simulink model "my_simulink_demo"  (Simulink 7.9)
settings: Solver=FixedStepDiscrete  StartTime=0.0  StopTime=0.0  RelTol=1e-3
undefined symbols (not defined in the file or in its folder): jet
libraries: visionsinks x3, visionanalysis x1, visionsources x1, visiongeotforms x1
settings Model: Creator=lenovo  LastModifiedBy=lenovo

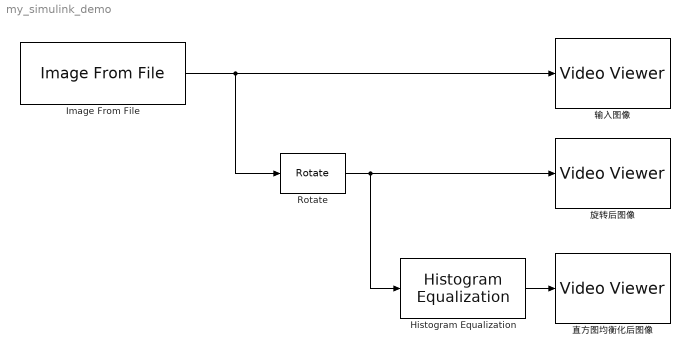
== system my_simulink_demo ==
  Histogram Equalization : visionanalysis/Histogram Equalization  specify=Uniform  numbins=64  src=Specify via dialog  hist=ones(1,64)
  Image From File : visionsources/Image From File  Tag=vipblks_nd  FileName=pout.tif  imagePorts=One multidimensional signal  Ts=inf  ImageDataType=Inherit from input image  Signed=on  WordLength=16  sdImageDataType=uint(8)  FractionLengthMode=User-defined  FractionLength=15  OutPortLabels=R|G|B
  Rotate : visiongeotforms/Rotate  outSizeR=Expanded to fit rotated input image  src_angle=Specify via dialog  unit_angle=Degrees  angle=pi/6  maxAngle=pi  dispImage=Center  method=Table lookup  fillVal=0  interpMethod=Bilinear  prodOutputMode=Binary point scaling  prodOutputWordLength=32  prodOutputFracLength=10  roundingMode=Nearest  overflowMode=on
  旋转后图像 : visionsinks/Video Viewer  inputType=Obsolete7b  imagePorts=One multidimensional signal  useColorMap=off  colormapValue=jet(256)  specRange=off  minInputVal=0  maxInputVal=255  FigPos=[812 550 410 300]  AxisZoom=on  trueSizedOnce=off  OpenAtMdlStart=on
  直方图均衡化后图像 : visionsinks/Video Viewer  inputType=Obsolete7b  imagePorts=One multidimensional signal  useColorMap=off  colormapValue=jet(256)  specRange=off  minInputVal=0  maxInputVal=255  FigPos=[111 514 410 300]  AxisZoom=on  trueSizedOnce=off  OpenAtMdlStart=on
  输入图像 : visionsinks/Video Viewer  inputType=Obsolete7b  imagePorts=One multidimensional signal  useColorMap=off  colormapValue=jet(256)  specRange=off  minInputVal=0  maxInputVal=255  FigPos=[440 617 410 300]  AxisZoom=on  trueSizedOnce=off  OpenAtMdlStart=on
  wires:
  Image From File/1 -> 输入图像/1, Rotate/1
  Rotate/1 -> 旋转后图像/1, Histogram Equalization/1
  Histogram Equalization/1 -> 直方图均衡化后图像/1
